simulink model "sample"  (R2018b)
settings: Solver=VariableStepAuto  StartTime=0.0  StopTime=0.0175  RelTol=1e-4
libraries: elec_lib x9, nesl_utility x8, fl_lib x3, pe_lib x1, pePwmGenerator x1, powerlib_meascontrol x1
settings Model: Creator=Shaun Zacharia  LastModifiedBy=Shaun Zacharia
settings SolverCC: ZeroCrossAlgorithm=Adaptive
settings DebuggingCC: MaskedZcDiagnostic=none  IgnoredZcDiagnostic=none

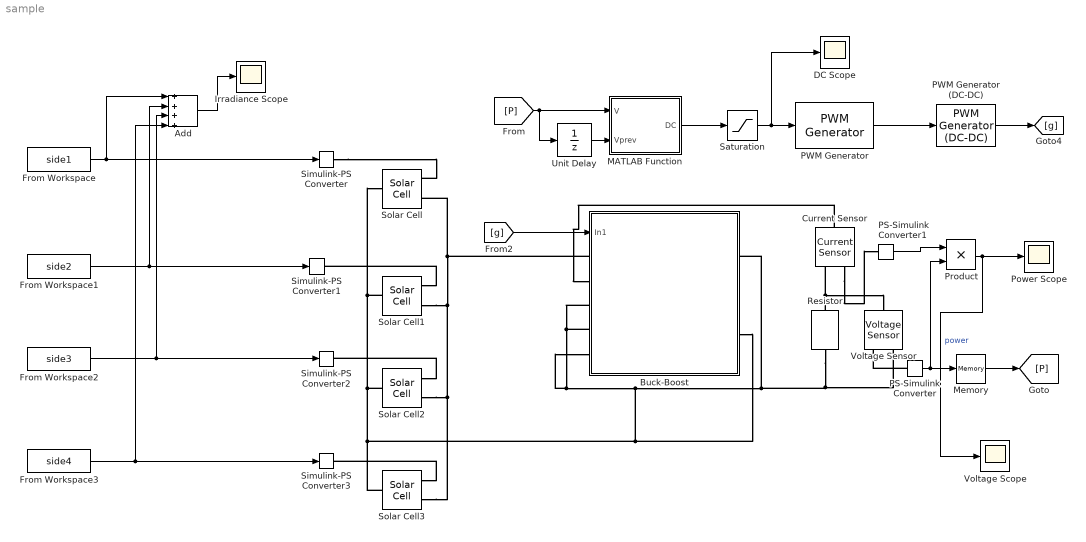
== system sample ==
  Add : Sum  Inputs=++++
  Buck-Boost : Subsystem
  Current Sensor : fl_lib/Electrical/Electrical Sensors/Current Sensor
  DC Scope : Scope
  From Workspace : FromWorkspace  VariableName=side1  SampleTime=0
  From Workspace1 : FromWorkspace  VariableName=side2  SampleTime=0
  From Workspace2 : FromWorkspace  VariableName=side3  SampleTime=0
  From Workspace3 : FromWorkspace  VariableName=side4  SampleTime=0
  Irradiance Scope : Scope
  MATLAB Function : MATLAB Function  TreatAsAtomicUnit=on
  Memory : Memory
  PS-Simulink Converter : nesl_utility/PS-Simulink Converter  PhysicalDomain=network_engine_domain  SubClassName=ps_output  LeftPortType=input  RightPortType=output  PseudoPeriodic=off  Frequencies=[]  Unit=1  AffineConversion=off
  PS-Simulink Converter1 : nesl_utility/PS-Simulink Converter  PhysicalDomain=network_engine_domain  SubClassName=ps_output  LeftPortType=input  RightPortType=output  PseudoPeriodic=off  Frequencies=[]  Unit=1  AffineConversion=off
  PWM Generator : pePwmGenerator/PWM Generator  CarrCount=Up  Tper=0.00001  Ts=0
  PWM Generator (DC-DC) : powerlib_meascontrol/Pulse & Signal Generators/PWM Generator (DC-DC)  Fsw=10e3  Ts=0
      settings: SourceProductName=Simscape Electrical
  Power Scope : Scope
  Product : Product
  Resistor : elec_lib/Passive Devices/Resistor  R=4.5 Ohm  R_tol=5  enable_R_tol=0  tol_distribution=1  nSigma=4  enable_operating_limits=0  operating_limit_action=2  max_working_voltage=100 V  power_rating=1 W  enable_faults=0  fault_action=1  R_faulted=inf Ohm  enable_temporal_fault=0  t_fault=1 s  enable_behavioral_fault=0  max_permissible_current=1 A  t_fail_on_current=1 s  noise_mode=0  sample_time=1e-3 s  repeatability=1  auto_seed=367287552  user_seed=0  Tdevice=25 degC  alpha=3.93e-3 1/K  Tmeas=25 degC  thermal_mass=100 J/K  power_derating_T1=70 degC  power_derating_T2=155 degC  operating_temperature_range_vec=[-50, 150] degC  temperature_specify=off  temperature_priority=High  temperature=298.15 K  temperature_nominal_specify=off  temperature_nominal_unit=K  temperature_nominal_value=1
  Saturation : Saturate  UpperLimit=1  LowerLimit=0
  Simulink-PS Converter{,1..3} (4 alike) : nesl_utility/Simulink-PS Converter  PhysicalDomain=network_engine_domain  SubClassName=ps_input  LeftPortType=input  RightPortType=output  PseudoPeriodic=off  Frequencies=[]  NoiseDistribution=none  NoiseParameters=[]  Unit=1  AffineConversion=off  FilteringAndDerivatives=provide  SimscapeFilterOrder=1  InputFilterTimeConstant=0.001  UdotUserProvided=0
  Solar Cell{,1..3} (4 alike) : elec_lib/Sources/Solar Cell  prm=1  Isc=0.5202 A  Voc=2.7 V  Is=1e-6 A  Is2=0 A  Iph=7.34 A  Ir0=1000 W/m^2  ec=1.5  N2=2  Rs=0 Ohm  Rp=inf Ohm  N_series=100  TIPH1=0 1/K  EG=1.11 eV  TXIS1=3  TXIS2=3  TRS1=0  TRP1=0  Tmeas=27 degC  TFIXED=27 degC  thermal_mass=100 J/K  initial_temperature=25 degC
      settings: SourceProductName=Simscape Electronics  SourceProductBaseCode=SN
  Unit Delay : UnitDelay  SampleTime=-1
  Voltage Scope : Scope
  Voltage Sensor : fl_lib/Electrical/Electrical Sensors/Voltage Sensor
  wires:
  From Workspace/1 -> Add/1, Simulink-PS Converter/1
  From Workspace1/1 -> Add/2, Simulink-PS Converter1/1
  From Workspace2/1 -> Add/3, Simulink-PS Converter2/1
  From Workspace3/1 -> Simulink-PS Converter3/1, Add/4
  PWM Generator/1 -> PWM Generator (DC-DC)/1
  MATLAB Function/1(DC) -> Saturation/1
  [P] -> MATLAB Function/1(V), Unit Delay/1
  Saturation/1 -> DC Scope/1, PWM Generator/1
  PWM Generator (DC-DC)/1 -> [g]
  [g] -> Buck-Boost/1(In1)
  PS-Simulink Converter/1 -> Product/2, Voltage Scope/1
  PS-Simulink Converter1/1 -> Product/1
  Product/1 -> Memory/1, Power Scope/1  "power"
  Memory/1 -> [P]
  Unit Delay/1 -> MATLAB Function/2(Vprev)
  Add/1 -> Irradiance Scope/1
  connections:
  Simulink-PS Converter/RConn1 -- Solar Cell/LConn1
  Solar Cell1/LConn1 -- Simulink-PS Converter1/RConn1
  Solar Cell2/LConn1 -- Simulink-PS Converter2/RConn1
  Solar Cell3/LConn1 -- Simulink-PS Converter3/RConn1
  Solar Cell2/LConn2 -- Solar Cell3/LConn2 -- Solar Cell1/LConn2 -- Buck-Boost/LConn1 -- Solar Cell/LConn2
  Buck-Boost/LConn4 -- Buck-Boost/LConn3 -- Buck-Boost/RConn2 -- Solar Cell3/RConn1 -- Solar Cell2/RConn1 -- Solar Cell1/RConn1 -- Solar Cell/RConn1 -- Resistor/RConn1 -- Voltage Sensor/RConn2 -- Buck-Boost/RConn1 -- Buck-Boost/LConn5
  Current Sensor/LConn1 -- Buck-Boost/LConn2
  Resistor/LConn1 -- Voltage Sensor/LConn1 -- Current Sensor/RConn2
  PS-Simulink Converter/LConn1 -- Voltage Sensor/RConn1
  Current Sensor/RConn1 -- PS-Simulink Converter1/LConn1

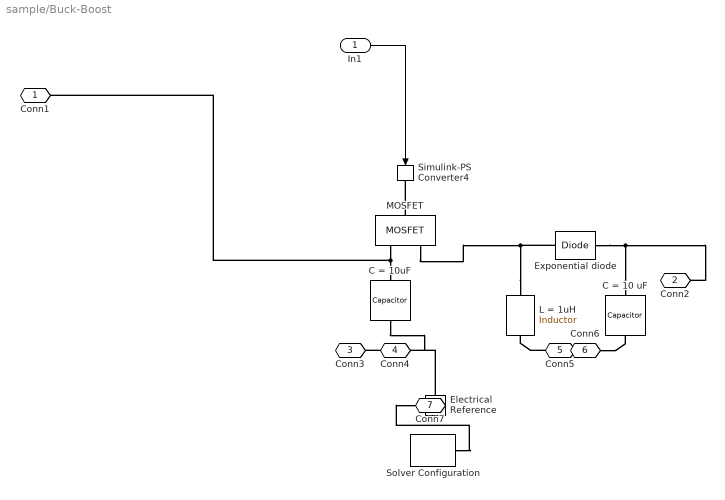
== system sample/Buck-Boost ==
  In1 : Inport
  C = 10 uF : elec_lib/Passive Devices/Capacitor  enable_table=0  c=10e-6 F  Cvec=[1e-05, 1e-06] F  Vvec=[0, 10] V  CV_table_symmetry=1  C_tol=5  enable_C_tol=0  tol_distribution=1  nSigma=4  r=0 Ohm  g=0 1/Ohm  enable_operating_limits=0  operating_limit_action=2  max_working_voltage_range=[-25, 25] V  power_rating=1 W  enable_faults=0  fault_action=1  Cscale_faulted=100  R_faulted=1e-3 Ohm  G_faulted=0 1/Ohm  tau_fault=1e-3 s  enable_temporal_fault=0  t_fault=1 s  enable_behavioral_fault=0  max_permissible_voltage_range=[-100, 100] V  t_fail_on_voltage=1 s  i_specify=off  i_priority=None  i=0 A  i_nominal_specify=off  i_nominal_unit=A  i_nominal_value=1  v_specify=off  v_priority=None  v=0 V  v_nominal_specify=off  v_nominal_unit=V  v_nominal_value=1  vc_specify=off  vc_priority=High  vc=0 V  vc_nominal_specify=off  vc_nominal_unit=V  vc_nominal_value=1
  C = 10uF : elec_lib/Passive Devices/Capacitor  enable_table=0  c=10e-6 F  Cvec=[1e-05, 1e-06] F  Vvec=[0, 10] V  CV_table_symmetry=1  C_tol=3  enable_C_tol=0  tol_distribution=1  nSigma=4  r=0 Ohm  g=0 1/Ohm  enable_operating_limits=0  operating_limit_action=2  max_working_voltage_range=[-25, 25] V  power_rating=1 W  enable_faults=0  fault_action=1  Cscale_faulted=100  R_faulted=1e-3 Ohm  G_faulted=0 1/Ohm  tau_fault=1e-3 s  enable_temporal_fault=0  t_fault=1 s  enable_behavioral_fault=0  max_permissible_voltage_range=[-100, 100] V  t_fail_on_voltage=1 s  i_specify=off  i_priority=None  i=0 A  i_nominal_specify=off  i_nominal_unit=A  i_nominal_value=1  v_specify=off  v_priority=None  v=0 V  v_nominal_specify=off  v_nominal_unit=V  v_nominal_value=1  vc_specify=off  vc_priority=High  vc=0 V  vc_nominal_specify=off  vc_nominal_unit=V  vc_nominal_value=1
  Electrical Reference : fl_lib/Electrical/Electrical Elements/Electrical Reference
  Exponential diode : elec_lib/Semiconductor Devices/Diode  ModelType=3  Vf=0.6 V  Ron=0.3 Ohm  Goff=1e-8 S  Rz=0.3 Ohm  Vz=50 V  C_PWL=5 pF  prmExp=1  I12=[.0137, .545] A  V12=[.6, .7] V  I1=0.0137 A  V1=0.6 V  IS=1e-12 A  ec=1  RS=0.01 Ohm  Tmeas=25 degC  BV=inf V  C_param=1  CJ0=5 pF  VJ=1 V  Mgrad=0.5  Vvec=[.1, 10, 100] V  Cvec=[3.5, 1, .4] pF  FC=0.5  Q_param=1  Irrm=-7.15 A  iF=4 A  didt=-750 A/us  trr=115 ns  TT=50 ns  tau=100 ns  T_param=1  IS_T2=1.25e-7 A  I1_T2=0.245 A  V1_T2=0.5 V  Tmeas2=125 degC  EG_param=1  EG=1.11 eV  XTI_param=1  XTI=3  dBVdT=0 V/K  Tdevice=25 degC  i_capacitor_specify=off  i_capacitor_priority=High  i_capacitor=0 A  i_capacitor_nominal_specify=off  i_capacitor_nominal_unit=A  i_capacitor_nominal_value=1  v_capacitor_specify=off  v_capacitor_priority=None  v_capacitor=0 V  v_capacitor_nominal_specify=off  v_capacitor_nominal_unit=V  v_capacitor_nominal_value=1  Rth=[0, 10] K/W  thermal_mass_parameterization=1  thermal_mass=[0, 1] J/K  thermal_time_constant=[0, 10] s  thermal_mass_initial_temperatures=[25, 25] degC
      settings: SourceProductName=Simscape Electronics  SourceProductBaseCode=SN
  L = 1uH : elec_lib/Passive Devices/Inductor  l=1e-6 H  L_tol=18  enable_L_tol=0  tol_distribution=1  nSigma=4  r=0.001 Ohm  g=1e-9 1/Ohm  enable_operating_limits=0  operating_limit_action=2  max_working_current=1 A  power_rating=1 W  enable_faults=0  fault_action=1  lambdaPercent=50  k_faulted=0.9999  turnsShort=0  openCct=0  groundShort=0  groundShortG=0 1/Ohm  tau_fault=1e-3 s  enable_temporal_fault=0  t_fault=1 s  enable_behavioral_fault=0  max_permissible_voltage=100 V  n_fail_on_voltage=1  max_permissible_current=1 A  t_fail_on_current=1 s  i_L_specify=off  i_L_priority=High  i_L=0 A  i_L_nominal_specify=off  i_L_nominal_unit=A  i_L_nominal_value=1
      settings: SourceProductName=Simscape Electronics  SourceProductBaseCode=SN
  MOSFET : pe_lib/Semiconductors/Fundamental Components/MOSFET  Rds=0.01 Ohm  Goff=1e-6 1/Ohm  Vth=0.5 V  diode_param=2  diode_Vf=0.8 V  diode_Ron=0.001 Ohm  diode_Goff=1e-5 1/Ohm  diode_C=5e-8 F  diode_iRM=-235 A  diode_iF=300 A  diode_idot=-50 A/us  diode_trr_param=1  diode_trr_factor=3  diode_trr=15 us  diode_Qrr=1.5e+3 s*uA  thermal_loss_option=2  Voff=300 V  Tau=1e-4 s  Tj=[ 298.15 398.15 ] K  Iout_scalar=600 A  Eon_scalar=0.02286 J  Eoff_scalar=0.01714 J  Von_scalar=2.7 V  Iout_data=[ 0 10 50 100 200 400 600 ] A  Eon_data=[ 0 2.9e-4 0.00143 0.00286 0.00571 0.01314 0.02286; 0 5.7e-4 0.00263 0.00514 0.01029 0.02057 0.03029 ] J  Eoff_data=[ 0 2.1e-4 0.00107 0.00214 0.00429 0.009859999999999999 0.01714; 0 4.3e-4 0.00197 0.00386 0.00771 0.01543 0.02271 ] J  Von_data=[ 0 1.1 1.3 1.45 1.75 2.25 2.7; 0 1 1.15 1.35 1.7 2.35 3 ] V
      settings: SourceProductName=Simscape Power Systems  SourceProductBaseCode=PS
  Simulink-PS Converter4 : nesl_utility/Simulink-PS Converter  PhysicalDomain=network_engine_domain  SubClassName=ps_input  LeftPortType=input  RightPortType=output  PseudoPeriodic=off  Frequencies=[]  NoiseDistribution=none  NoiseParameters=[]  Unit=1  AffineConversion=off  FilteringAndDerivatives=provide  SimscapeFilterOrder=1  InputFilterTimeConstant=0.001  UdotUserProvided=0
  Solver Configuration : nesl_utility/Solver Configuration  PhysicalDomain=network_engine_domain  SubClassName=solver  LeftPortType=input  RightPortType=generic  Tones=[]  Harmonics=[]  SimulateNoise=off  Profile=off  UseLocalSampling=off  EnableSwitchedLinearOptims=on  FrequencyDomain=off  UseCCode=off  RelTol=0.001  AbsTol=1e-06  MinStep=1e-09  ToWorkspace=off  RevertToSquareIcSolve=off  NumHomotopyIterations=100  PhasorMode=off  PhasorModeNumHarmonics=1  DoDC=off  ResidualTolerance=1e-09  UseLocalSolver=off  LocalSolverChoice=NE_BACKWARD_EULER_ADVANCER  LocalSolverSampleTime=0.001  DoFixedCost=off  MaxNonlinIter=3  MaxModeIter=2  LinearAlgebra=auto  EquationFormulation=NE_TIME_EF  DelaysMemoryBudget=1024  AutomaticFiltering=on  FilteringTimeConstant=0.001  PartitionStorageMethod=AS_NEEDED  PartitionMemoryBudget=1024
  Conn1 : PMIOPort  Side=Left
  Conn2 : PMIOPort  Port=2  Side=Left
  Conn3 : PMIOPort  Port=3  Side=Left
  Conn4 : PMIOPort  Port=4  Side=Left
  Conn5 : PMIOPort  Port=5  Side=Right
  Conn6 : PMIOPort  Port=6  Side=Left
  Conn7 : PMIOPort  Port=7  Side=Right
  wires:
  In1/1 -> Simulink-PS Converter4/1
  connections:
  Conn6/RConn1 -- C = 10 uF/LConn1
  L = 1uH/LConn1 -- MOSFET/RConn2 -- Exponential diode/RConn1
  C = 10uF/LConn1 -- Conn3/RConn1
  C = 10 uF/RConn1 -- Exponential diode/LConn1 -- Conn2/RConn1
  MOSFET/RConn1 -- Conn1/RConn1 -- C = 10uF/RConn1
  Electrical Reference/LConn1 -- Conn4/RConn1
  MOSFET/LConn1 -- Simulink-PS Converter4/RConn1
  Solver Configuration/RConn1 -- Conn7/RConn1
  Conn5/RConn1 -- L = 1uH/RConn1

== matlab function sample/MATLAB Function ==
  settings: updateMethod=DISCRETE
  data: V input; DC output; Vprev input
function DC = fcn(V, Vprev)

persistent DCprev DCnew
incDC = 0.001;
% The amout by which it will be changed each time; equivalent to 1%

if isempty(DCprev)
    DCprev = 0.1;
    DCnew = 0.12;
else
    DC = DCnew;
end

if V ~= Vprev 
    if V > Vprev
        if DCnew > DCprev
            DCprev = DCnew;
            DCnew = DCnew + incDC;
            DC = DCnew;
        else
            DCprev = DCnew;
            DCnew = DCnew - incDC;
            DC = DCnew;
        end
    else
        if DCnew > DCprev
            DCprev = DCnew;
            DCnew = DCprev - incDC;
            DC = DCnew;
        else
            DCprev = DCnew;
            DCnew = DCprev + incDC;
            DC = DCnew;
        end
    end
else
    DCnew = DCprev;
    DC = DCnew;
end

Pprev = V;
% update the values.
